simulink model "Force_Att_Controller_Separated"  (R2020a)
settings: Solver=FixedStepAuto  StartTime=0.0  StopTime=20  FixedStep=P.Ts  RelTol=1e-3
PreLoadFcn:
  | parameters
values from neighbouring files (symbols this model uses):
  beta1 = 1    [Run_force_Att_Controller.m]
  kTheta = 0.5/N    (= 0.00333333333333)    [Run_force_Att_Controller.m]
  L = 3    [Run_force_Att_Controller.m]
  m = 3    [Run_force_Att_Controller.m]
  n = length(q)    [Run_force_Att_Controller.m]    (also in circlePoints.m = numberOfPoints)
  N = 150    [Run_force_Att_Controller.m]
  T1 = 1    [Run_force_Att_Controller.m]
  T2 = 0.6    [Run_force_Att_Controller.m]
  ThetaHat0 = [ones(9,1)*1;1]    [Run_force_Att_Controller.m]
  ThetaStar = [0.2061;0.2061;0.2061;0.2061;0.2061;0.2061;6.7315;2.6926;0;1.5]    [Run_force_Att_Controller.m]
  Ts = P.Ts    [Run_force_Att_Controller.m]
  x1_int = [0;-0.15;0.5]    [Run_force_Att_Controller.m]
  x1Dot = [0;0;0]    [Run_force_Att_Controller.m]
  x2_int = [0;0.15;0.5]    [Run_force_Att_Controller.m]
  x2Dot = [0;0;0]    [Run_force_Att_Controller.m]
  xc_int = [0;0;0.5]    [Run_force_Att_Controller.m]
  xcDot = [0;0;0]    [Run_force_Att_Controller.m]
undefined symbols (not defined in the file or in its folder): P
(part 1 of 2)
settings Model: Creator=Daslab  LastModifiedBy=thapa
settings DataIOCC: ReturnWorkspaceOutputs=off
settings DebuggingCC: ArithmeticOperatorsInVariantConditions=warning
settings SFSimCC: SimUseLocalCustomCode=off  CustomCodeUndefinedFunction=UseInterfaceOnly
settings RTWCC: RTWUseLocalCustomCode=off

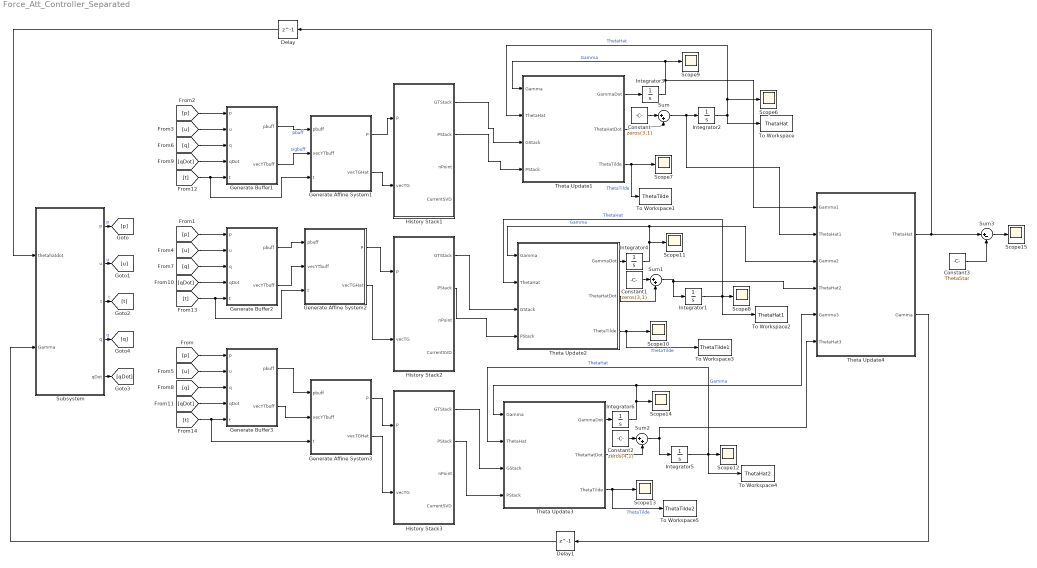
== system Force_Att_Controller_Separated ==
  Constant : Constant  Value=zeros(3,1)
  Constant1 : Constant  Value=zeros(3,1)
  Constant2 : Constant  Value=zeros(4,1)
  Constant3 : Constant  Value=ThetaStar
  Delay : Delay  DelayLength=1  InitialCondition=0
  Delay1 : Delay  DelayLength=1  InitialCondition=0
  Generate Affine System1 : MATLAB Function  TreatAsAtomicUnit=on
  Generate Affine System2 : MATLAB Function  TreatAsAtomicUnit=on
  Generate Affine System3 : MATLAB Function  TreatAsAtomicUnit=on
  Generate Buffer1 : MATLAB Function  TreatAsAtomicUnit=on
  Generate Buffer2 : MATLAB Function  TreatAsAtomicUnit=on
  Generate Buffer3 : MATLAB Function  TreatAsAtomicUnit=on
  History Stack1 : MATLAB Function  TreatAsAtomicUnit=on
  History Stack2 : MATLAB Function  TreatAsAtomicUnit=on
  History Stack3 : MATLAB Function  TreatAsAtomicUnit=on
  Integrator1 : Integrator  InitialCondition=ThetaHat0(4:6,1)
  Integrator2 : Integrator  InitialCondition=ThetaHat0(1:3,1)
  Integrator3 : Integrator  InitialCondition=eye(3)
  Integrator4 : Integrator  InitialCondition=eye(3)
  Integrator5 : Integrator  InitialCondition=ThetaHat0(7:10,1)
  Integrator6 : Integrator  InitialCondition=eye(4)
  Scope{6..15} (10 alike) : Scope
  Subsystem : Subsystem
  Sum : Sum  Inputs=|++
  Sum1 : Sum  Inputs=|++
  Sum2 : Sum  Inputs=|++
  Sum3 : Sum  Inputs=|+-
  Theta Update1 : MATLAB Function  TreatAsAtomicUnit=on
  Theta Update2 : MATLAB Function  TreatAsAtomicUnit=on
  Theta Update3 : MATLAB Function  TreatAsAtomicUnit=on
  Theta Update4 : MATLAB Function  TreatAsAtomicUnit=on
  To Workspace : ToWorkspace  VariableName=ThetaHat  SaveFormat=Timeseries  SampleTime=-1
  To Workspace1 : ToWorkspace  VariableName=ThetaTilde  SaveFormat=Timeseries  SampleTime=-1
  To Workspace2 : ToWorkspace  VariableName=ThetaHat1  SaveFormat=Timeseries  SampleTime=-1
  To Workspace3 : ToWorkspace  VariableName=ThetaTilde1  SaveFormat=Timeseries  SampleTime=-1
  To Workspace4 : ToWorkspace  VariableName=ThetaHat2  SaveFormat=Timeseries  SampleTime=-1
  To Workspace5 : ToWorkspace  VariableName=ThetaTilde2  SaveFormat=Timeseries  SampleTime=-1
  wires:
  Theta Update1/3(ThetaTilde) -> Scope7/1, To Workspace1/1  "ThetaTilde"
  History Stack1/1(GTStack) -> Theta Update1/3(GStack)
  Generate Affine System1/1(P) -> History Stack1/1(P)
  Integrator2/1 -> Scope6/1, Theta Update1/2(ThetaHat), To Workspace/1  "ThetaHat"
  History Stack1/2(PStack) -> Theta Update1/4(PStack)
  Integrator3/1 -> Scope9/1, Theta Update1/1(Gamma), Theta Update4/1(Gamma1)  "Gamma"
  Theta Update1/1(GammaDot) -> Integrator3/1
  Constant/1 -> Sum/1
  Sum/1 -> Theta Update4/2(ThetaHat1), Integrator2/1
  Theta Update1/2(ThetaHatDot) -> Sum/2
  Delay/1 -> Subsystem/1(thetahatdot)
  Generate Buffer1/1(pbuff) -> Generate Affine System1/1(pbuff)  "pbuff"
  Generate Buffer1/2(vecYTbuff) -> Generate Affine System1/2(vecYTbuff)  "sigbuff"
  Generate Affine System1/2(vecTGHat) -> History Stack1/2(vecTG)
  History Stack2/1(GTStack) -> Theta Update2/3(GStack)
  History Stack2/2(PStack) -> Theta Update2/4(PStack)
  History Stack3/1(GTStack) -> Theta Update3/3(GStack)
  History Stack3/2(PStack) -> Theta Update3/4(PStack)
  Sum1/1 -> Theta Update4/4(ThetaHat2), Integrator1/1
  Theta Update2/2(ThetaHatDot) -> Sum1/2
  Integrator4/1 -> Scope11/1, Theta Update4/3(Gamma2), Theta Update2/1(Gamma)  "Gamma"
  Constant1/1 -> Sum1/1
  Integrator1/1 -> Theta Update2/2(ThetaHat), Scope8/1, To Workspace2/1  "ThetaHat"
  Theta Update2/3(ThetaTilde) -> Scope10/1, To Workspace3/1  "ThetaTilde"
  Theta Update2/1(GammaDot) -> Integrator4/1
  Sum2/1 -> Theta Update4/6(ThetaHat3), Integrator5/1
  Theta Update3/2(ThetaHatDot) -> Sum2/2
  Integrator6/1 -> Scope14/1, Theta Update3/1(Gamma), Theta Update4/5(Gamma3)  "Gamma"
  Constant2/1 -> Sum2/1
  Integrator5/1 -> Theta Update3/2(ThetaHat), Scope12/1, To Workspace4/1  "ThetaHat"
  Theta Update3/3(ThetaTilde) -> Scope13/1, To Workspace5/1  "ThetaTilde"
  Theta Update3/1(GammaDot) -> Integrator6/1
  Generate Affine System3/1(P) -> History Stack3/1(P)
  Generate Affine System3/2(vecTGHat) -> History Stack3/2(vecTG)
  Generate Affine System2/1(P) -> History Stack2/1(P)
  Generate Affine System2/2(vecTGHat) -> History Stack2/2(vecTG)
  Generate Buffer2/1(pbuff) -> Generate Affine System2/1(pbuff)
  Generate Buffer2/2(vecYTbuff) -> Generate Affine System2/2(vecYTbuff)
  Generate Buffer3/1(pbuff) -> Generate Affine System3/1(pbuff)
  Generate Buffer3/2(vecYTbuff) -> Generate Affine System3/2(vecYTbuff)
  Theta Update4/2(Gamma) -> Delay1/1
  Delay1/1 -> Subsystem/2(Gamma)
  Theta Update4/1(ThetaHat) -> Sum3/1, Delay/1
  Constant3/1 -> Sum3/2
  Sum3/1 -> Scope15/1
  Subsystem/1(p) -> [p]  "p"
  [p] -> Generate Buffer1/1(p)
  Subsystem/2(u) -> [u]  "u"
  Subsystem/5(qDot) -> [qDot]
  Subsystem/4(q) -> [q]  "q"
  Subsystem/3(t) -> [t]  "t"
  [p] -> Generate Buffer2/1(p)
  [p] -> Generate Buffer3/1(p)
  [u] -> Generate Buffer1/2(u)
  [u] -> Generate Buffer2/2(u)
  [u] -> Generate Buffer3/2(u)
  [q] -> Generate Buffer1/3(q)
  [q] -> Generate Buffer2/3(q)
  [q] -> Generate Buffer3/3(q)
  [qDot] -> Generate Buffer1/4(qDot)
  [qDot] -> Generate Buffer2/4(qDot)
  [qDot] -> Generate Buffer3/4(qDot)
  [t] -> Generate Affine System1/3(t), Generate Buffer1/5(t)
  [t] -> Generate Affine System2/3(t), Generate Buffer2/5(t)
  [t] -> Generate Affine System3/3(t), Generate Buffer3/5(t)

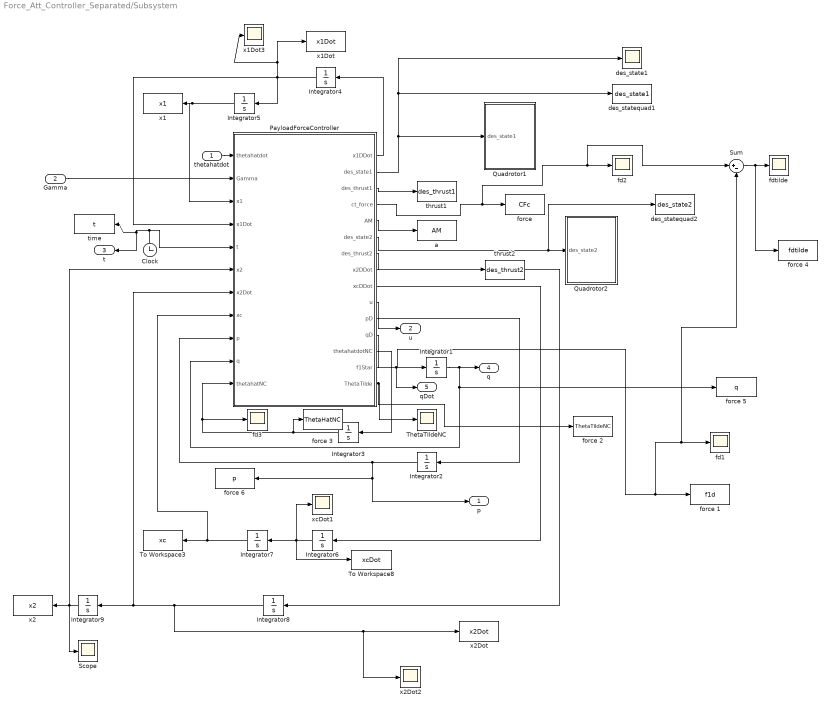
== system Force_Att_Controller_Separated/Subsystem ==
  thetahatdot : Inport
  Gamma : Inport  Port=2
  Clock : Clock
  Integrator1 : Integrator  InitialCondition=[x1Dot;x2Dot;xcDot]
  Integrator2 : Integrator  InitialCondition=[x1_int;x2_int;xc_int]
  Integrator3 : Integrator  InitialCondition=ones(10,1)
  Integrator4 : Integrator  InitialCondition=x1Dot
  Integrator5 : Integrator  InitialCondition=x1_int
  Integrator6 : Integrator  InitialCondition=xcDot
  Integrator7 : Integrator  InitialCondition=xc_int
  Integrator8 : Integrator  InitialCondition=x2Dot
  Integrator9 : Integrator  InitialCondition=x2_int
  PayloadForceController : MATLAB Function  TreatAsAtomicUnit=on
  Quadrotor1 : Subsystem
  Quadrotor2 : Subsystem
  Scope : Scope
  Sum : Sum  Inputs=|+-
  ThetaTIldeNC : Scope
  To Workspace3 : ToWorkspace  VariableName=xc  SampleTime=-1
  To Workspace8 : ToWorkspace  VariableName=xcDot  SampleTime=-1
  "a " : ToWorkspace  VariableName=AM  SampleTime=-1
  des_state1 : Scope
  "des_statequad1 " : ToWorkspace  VariableName=des_state1  SampleTime=-1
      settings: Save2DSignal=2-D array (concatenate along first dimension)
  des_statequad2 : ToWorkspace  VariableName=des_state2  SampleTime=-1
      settings: Save2DSignal=2-D array (concatenate along first dimension)
  fd1 : Scope
  fd2 : Scope
  fd3 : Scope
  fdtilde : Scope
  "force " : ToWorkspace  VariableName=CFc  SampleTime=-1
  force 1 : ToWorkspace  VariableName=f1d  SampleTime=-1
  force 2 : ToWorkspace  VariableName=ThetaTildeNC  SampleTime=-1
  force 3 : ToWorkspace  VariableName=ThetaHatNC  SampleTime=-1
  force 4 : ToWorkspace  VariableName=fdtilde  SampleTime=-1
  force 5 : ToWorkspace  VariableName=q  SampleTime=-1
      settings: Save2DSignal=2-D array (concatenate along first dimension)
  force 6 : ToWorkspace  VariableName=p  SampleTime=-1
      settings: Save2DSignal=2-D array (concatenate along first dimension)
  thrust1 : ToWorkspace  VariableName=des_thrust1  SampleTime=-1
      settings: Save2DSignal=2-D array (concatenate along first dimension)
  thrust2 : ToWorkspace  VariableName=des_thrust2  SampleTime=-1
  time : ToWorkspace  VariableName=t  SampleTime=-1
  x1 : ToWorkspace  VariableName=x1  SampleTime=-1
  x1Dot : ToWorkspace  VariableName=x1Dot  SampleTime=-1
  x1Dot3 : Scope
  x2 : ToWorkspace  VariableName=x2  SampleTime=-1
  x2Dot : ToWorkspace  VariableName=x2Dot  SampleTime=-1
  x2Dot2 : Scope
  xcDot1 : Scope
  p : Outport  VectorParamsAs1DForOutWhenUnconnected=off
  u : Outport  Port=2  VectorParamsAs1DForOutWhenUnconnected=off
  t : Outport  Port=3  VectorParamsAs1DForOutWhenUnconnected=off
  q : Outport  Port=4  VectorParamsAs1DForOutWhenUnconnected=off
  qDot : Outport  Port=5  VectorParamsAs1DForOutWhenUnconnected=off
  wires:
  PayloadForceController/7(des_thrust2) -> thrust2/1
  Integrator6/1 -> Integrator7/1, xcDot1/1, To Workspace8/1
  PayloadForceController/4(ct_force) -> Sum/1, fd2/1, "force "/1
  PayloadForceController/9(xcDDot) -> Integrator6/1
  PayloadForceController/5(AM) -> "a "/1
  PayloadForceController/2(des_state1) -> "des_statequad1 "/1, des_state1/1, Quadrotor1/1(des_state1)
  PayloadForceController/3(des_thrust1) -> thrust1/1
  Clock/1 -> time/1, t/1, PayloadForceController/5(t)
  Integrator7/1 -> PayloadForceController/8(xc), To Workspace3/1
  Integrator8/1 -> PayloadForceController/7(x2Dot), Integrator9/1, x2Dot2/1, x2Dot/1
  PayloadForceController/1(x1DDot) -> Integrator4/1
  Integrator4/1 -> Integrator5/1, x1Dot3/1, x1Dot/1, PayloadForceController/4(x1Dot)
  Integrator9/1 -> Scope/1, PayloadForceController/6(x2), x2/1
  Integrator5/1 -> PayloadForceController/3(x1), x1/1
  PayloadForceController/6(des_state2) -> des_statequad2/1, Quadrotor2/1(des_state2)
  PayloadForceController/8(x2DDot) -> Integrator8/1
  PayloadForceController/10(u) -> u/1
  Integrator1/1 -> PayloadForceController/10(q), force 5/1, q/1
  Integrator2/1 -> p/1, force 6/1, PayloadForceController/9(p)
  PayloadForceController/11(pD) -> Integrator2/1
  PayloadForceController/12(qD) -> qDot/1, Integrator1/1
  thetahatdot/1 -> PayloadForceController/1(thetahatdot)
  PayloadForceController/13(thetahatdotNC) -> Integrator3/1
  Integrator3/1 -> force 3/1, PayloadForceController/11(thetahatNC), fd3/1
  Gamma/1 -> PayloadForceController/2(Gamma)
  PayloadForceController/14(f1Star) -> Sum/2, fd1/1, force 1/1
  PayloadForceController/15(ThetaTilde) -> force 2/1, ThetaTIldeNC/1
  Sum/1 -> force 4/1, fdtilde/1

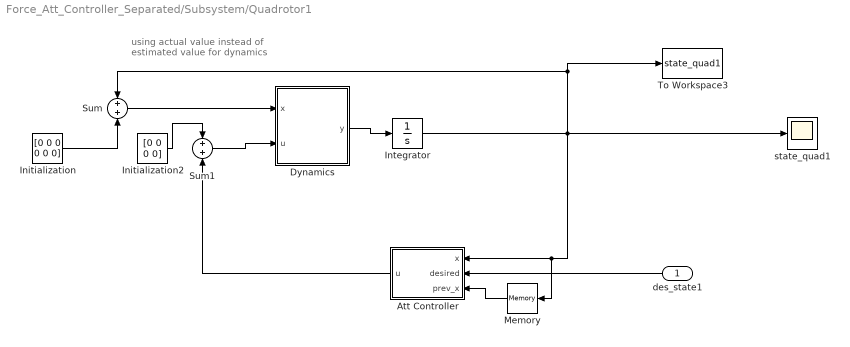
== system Force_Att_Controller_Separated/Subsystem/Quadrotor1 ==
  note: using actual value instead of estimated value for dynamics
  des_state1 : Inport
  Att Controller : MATLAB Function  TreatAsAtomicUnit=on
  Dynamics : MATLAB Function  TreatAsAtomicUnit=on  SystemSampleTime=P.Ts
  Initialization : Constant  Value=[0 0 0 0 0 0]
  Initialization2 : Constant  Value=[0 0 0 0]
  Integrator : Integrator
  Memory : Memory  InitialCondition=[0 0 0 0 0 0]
  Sum : Sum
  Sum1 : Sum
  To Workspace3 : ToWorkspace  VariableName=state_quad1  SampleTime=-1
      settings: Save2DSignal=2-D array (concatenate along first dimension)
  state_quad1 : Scope
  wires:
  Memory/1 -> Att Controller/3(prev_x)
  Initialization2/1 -> Sum1/1
  Att Controller/1(u) -> Sum1/2
  Dynamics/1(y) -> Integrator/1
  Initialization/1 -> Sum/2
  Integrator/1 -> Memory/1, Att Controller/1(x), state_quad1/1, Sum/1, To Workspace3/1
  Sum1/1 -> Dynamics/2(u)
  Sum/1 -> Dynamics/1(x)
  des_state1/1 -> Att Controller/2(desired)

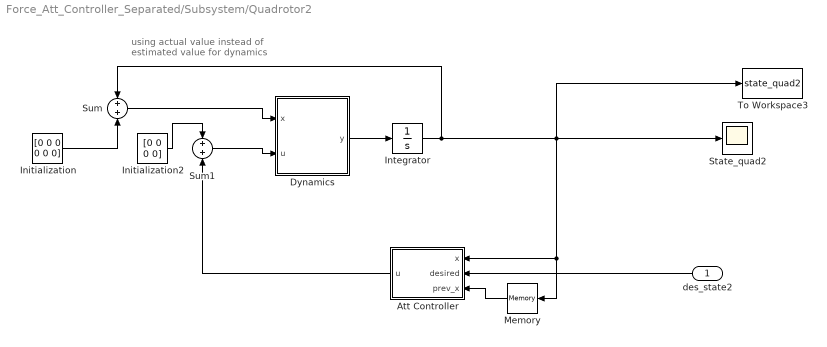
== system Force_Att_Controller_Separated/Subsystem/Quadrotor2 ==
  note: using actual value instead of estimated value for dynamics
  des_state2 : Inport
  Att Controller : MATLAB Function  TreatAsAtomicUnit=on
  Dynamics : MATLAB Function  TreatAsAtomicUnit=on  SystemSampleTime=P.Ts
  Initialization : Constant  Value=[0 0 0 0 0 0]
  Initialization2 : Constant  Value=[0 0 0 0]
  Integrator : Integrator
  Memory : Memory  InitialCondition=[0 0 0 0 0 0]
  State_quad2 : Scope
  Sum : Sum
  Sum1 : Sum
  To Workspace3 : ToWorkspace  VariableName=state_quad2  SampleTime=-1
      settings: Save2DSignal=2-D array (concatenate along first dimension)
  wires:
  Memory/1 -> Att Controller/3(prev_x)
  Initialization2/1 -> Sum1/1
  Att Controller/1(u) -> Sum1/2
  Dynamics/1(y) -> Integrator/1
  Initialization/1 -> Sum/2
  Integrator/1 -> State_quad2/1, Memory/1, Att Controller/1(x), To Workspace3/1, Sum/1
  Sum1/1 -> Dynamics/2(u)
  Sum/1 -> Dynamics/1(x)
  des_state2/1 -> Att Controller/2(desired)

== matlab function Force_Att_Controller_Separated/Subsystem/Quadrotor2/Dynamics ==
  data: x input; u input; y output; P parameter
function y = fcn(x, u, P)
%#codegen
%References: Quadrotor Dynamics and Control Rev 0.1
%Randal Beard

%A Simple Attitude Control of Quadrotor Helicopter Based on
%Ziegler-Nichols Rules for Tuning PD Parameters
%ZeFang He and Long Zhao

wind = [0 0 0]';

m = P.m;
g = P.g;
Ix = P.Ix;
Iy = P.Iy;
Iz = P.Iz;
L = P.L;

Cd = zeros(3,1);
Cd(1:3) = P.Cd1 + 0.9*exp(-0.6*(norm(wind(1:3)+x(4:6))-2));


% Cd = zeros(3,1);
% Cd(1) = P.Cd1 + 0.9*exp(-0.6*(abs(wind(1)+x(4)) - 2));
% Cd(2) = P.Cd2 + 0.9*exp(-0.6*(abs(wind(2)+x(5)) - 2));
% Cd(3) = P.Cd3 + 0.9*exp(-0.6*(abs(wind(3)+x(6)) - 2));
for i=1:3
    if Cd(i) > 1.1
        Cd(i) = 1.1;
    end
end

y = x;

%Calculate drag force on quadrotor
mag_V = wind + x(4:6);
%mag_V = x(4:6);
mag_Combined = norm(mag_V); %airspeed magnitude
force = Cd * mag_Combined^2;

Fw = zeros(3,1);
if mag_Combined ~= 0
    Fw = diag(mag_V/mag_Combined) * force;
else
    Fw(:) = 0;
end

% y(1) = -x(4) + wind(1);
% y(2) = -x(5) + (wind(2));
% y(3) = -x(6) + (wind(3));
%y(1) = 0;%-x(4);
%y(2) = 0;%-x(5);
%y(3) = 0;%-x(6);
%y(4) = 0;%(u(1))/m*(cos(x(7))*sin(x(8))*cos(x(9)) +...
    %sin(x(7))*sin(x(9))) + Fw(1)/m;%1/m*sign(x(4))*Cd1*x(4)^2;
%y(5) = 0;%-(u(1))/m*(+cos(x(7))*sin(x(8))*sin(x(9)) -...
    %sin(x(7))*cos(x(9))) + Fw(2)/m;%1/m*sign(x(5))*Cd2*x(5)^2;
%y(6) = 0;%g - (u(1))/m*(cos(x(7)) * cos(x(8))) + Fw(3);%1/m*sign(x(6))*Cd3*x(5)^2;

%roll, pitch, yaw: phi, theta, psi
y(1) = x(4);
y(2) = x(5);
y(3) = x(6);
y(4) = x(5)*x(6)*(Iy-Iz)/Ix + 1/Ix*u(2);
y(5) = x(4)*x(6)*(Iz-Ix)/Iy + 1/Iy*u(3);
y(6) = x(4)*x(5)*(Ix - Iy)/Iz + u(4)/Iz;

== matlab function Force_Att_Controller_Separated/Generate Buffer2 ==
  settings: updateMethod=DISCRETE  sampleTime=Ts
  data: pbuff output; p input; u input; q input; qDot input; t input; T1 parameter; T2 parameter; Ts parameter; n parameter; L parameter; vecYTbuff output; P parameter
function [pbuff,vecYTbuff] = fcn(p,u,q,qDot,t,T1,T2,Ts,n,L,P)
%#codegen
persistent PTemp sigTemp;
if isempty(PTemp)
    PTemp = 0*ones(n/3,round((T1)/Ts)+1); % initalize the persistent variable
end

if isempty(sigTemp)
    sigTemp = zeros(n/3*L,round((T1)/Ts)+1);
end
% Known part of the system dynamics
qDotbuff = zeros(9,1);
x1 = p(1:3,1);
x2 = p(4:6,1);
xc = p(7:9,1);
x1Dot = q(1:3,1);
x2Dot = q(4:6,1);
xcDot = q(7:9,1);
m1 = P.m;
m2 = m1;
Mc = P.Mc;
g = P.g;
k = P.k;

e3 = [0 0 1]';

R_theta = eye(3,3);     

r1 = [0 -0.15 0]';
r2 = [0 0.15 0]';

a1 = xc + R_theta*r1; 

a2 = xc + R_theta*r2;

z1 = x1 - a1;

z2 = x2 - a2;

f1 = k*z1;  % linear model 

f2 = k*z2;   % linear model 


fo = [(u(4:6,1) - f2 - m2*g*e3)/m2];

Y_N = diag([1/m2*norm(x2Dot)*x2Dot]);
Y_c = [eye(3),qDot(7:9,1) + g*e3];


Y = [Y_N];
 
qDotbuff(1:6,1) = qDot(1:6,1);
qDotbuff(7:9,1) = zeros(3,1);

sig = reshape(Y.',n/3*L,1);

PPP=PTemp(:,2:end);
SSS=sigTemp(:,2:end);
PTemp=[PPP fo-qDotbuff(4:6,1)];
sigTemp=[SSS sig];
pbuff=PTemp;
vecYTbuff=sigTemp;

== matlab function Force_Att_Controller_Separated/Generate Affine System2 ==
  data: P output; pbuff input; vecYTbuff input; t input; Ts parameter; T2 parameter; T1 parameter; vecTGHat output
function [P,vecTGHat]  = fcn(pbuff,vecYTbuff,t ,Ts, T2, T1)
%#codegen
T1Round=round(T1/Ts);

P1=pbuff(:,end-T1Round:end);
G1=vecYTbuff(:,end-T1Round:end);

P = (t>T1)*Ts*trapz(P1,2);
vecTGHat = (t>T1)*Ts*trapz(G1,2);

== matlab function Force_Att_Controller_Separated/Subsystem/Quadrotor1/Dynamics ==
  data: x input; u input; y output; P parameter
function y = fcn(x, u, P)
%#codegen
%References: Quadrotor Dynamics and Control Rev 0.1
%Randal Beard

%A Simple Attitude Control of Quadrotor Helicopter Based on
%Ziegler-Nichols Rules for Tuning PD Parameters
%ZeFang He and Long Zhao

wind = [0 0 0]';

m = P.m;
g = P.g;
Ix = P.Ix;
Iy = P.Iy;
Iz = P.Iz;
L = P.L;

Cd = zeros(3,1);
Cd(1:3) = P.Cd1 + 0.9*exp(-0.6*(norm(wind(1:3)+x(4:6))-2));


% Cd = zeros(3,1);
% Cd(1) = P.Cd1 + 0.9*exp(-0.6*(abs(wind(1)+x(4)) - 2));
% Cd(2) = P.Cd2 + 0.9*exp(-0.6*(abs(wind(2)+x(5)) - 2));
% Cd(3) = P.Cd3 + 0.9*exp(-0.6*(abs(wind(3)+x(6)) - 2));
for i=1:3
    if Cd(i) > 1.1
        Cd(i) = 1.1;
    end
end

y = x;

%Calculate drag force on quadrotor
mag_V = wind + x(4:6);
%mag_V = x(4:6);
mag_Combined = norm(mag_V); %airspeed magnitude
force = Cd * mag_Combined^2;

Fw = zeros(3,1);
if mag_Combined ~= 0
    Fw = diag(mag_V/mag_Combined) * force;
else
    Fw(:) = 0;
end

% y(1) = -x(4) + wind(1);
% y(2) = -x(5) + (wind(2));
% y(3) = -x(6) + (wind(3));
%y(1) = 0;%-x(4);
%y(2) = 0;%-x(5);
%y(3) = 0;%-x(6);
%y(4) = 0;%(u(1))/m*(cos(x(7))*sin(x(8))*cos(x(9)) +...
    %sin(x(7))*sin(x(9))) + Fw(1)/m;%1/m*sign(x(4))*Cd1*x(4)^2;
%y(5) = 0;%-(u(1))/m*(+cos(x(7))*sin(x(8))*sin(x(9)) -...
    %sin(x(7))*cos(x(9))) + Fw(2)/m;%1/m*sign(x(5))*Cd2*x(5)^2;
%y(6) = 0;%g - (u(1))/m*(cos(x(7)) * cos(x(8))) + Fw(3);%1/m*sign(x(6))*Cd3*x(5)^2;

%roll, pitch, yaw: phi, theta, psi
y(1) = x(4);
y(2) = x(5);
y(3) = x(6);
y(4) = x(5)*x(6)*(Iy-Iz)/Ix + 1/Ix*u(2);
y(5) = x(4)*x(6)*(Iz-Ix)/Iy + 1/Iy*u(3);
y(6) = x(4)*x(5)*(Ix - Iy)/Iz + u(4)/Iz;

== matlab function Force_Att_Controller_Separated/History Stack2 ==
  settings: updateMethod=DISCRETE  sampleTime=Ts
  data: P input; GTStack output; vecTG input; N parameter; n parameter; L parameter; PStack output; nPoint output; CurrentSVD output
function [GTStack,PStack,nPoint,CurrentSVD] =...
    fcn(P,vecTG, N, n, L )
%#codegen,FStackStored, GStackStored, PStackStored
persistent GStackHPersist PStackHPersist nPoints eta;
% if isempty(FStackHPersist)
% %    FStackHPersist = FStackStored; % initalize the persistent variable
%      FStackHPersist = zeros(n,N);
% end
if isempty(GStackHPersist)
 %   GStackHPersist = GStackStored;
    GStackHPersist = zeros(L,n/3*N);
end
if isempty(PStackHPersist)
%    PStackHPersist = PStackStored;
     PStackHPersist = zeros(n/3,N);
end
if isempty(nPoints)
    nPoints = 0;
end
if isempty(eta)
    eta = 0;
end
%GHatTStack is [intY1' intY2' ... intYN']
%FHatStack is [FHat1 FHat2 ... FHatN]
%and so is PStack
G = (reshape(vecTG,L,n/3)).';

%Operations 
CurrentScriptH = GStackHPersist*GStackHPersist';
CurrentSingularValue = min(svd(CurrentScriptH));
SingularValueList = zeros(N,1);
for i=1:N
    ithGTranspose = GStackHPersist(:,(i-1)*n/3+1:i*n/3);
    NewScriptH = CurrentScriptH + G'*G...
        -ithGTranspose*ithGTranspose';
    SingularValueList(i,1)=min(svd(NewScriptH));
end

[NewSingularValue,ind]=max(SingularValueList);
%Update persistent variables
if NewSingularValue>CurrentSingularValue + 0*CurrentSingularValue
    GStackHPersist(:,(ind-1)*n/3+1:ind*n/3) = G';
    %FStackHPersist(:,ind) = FHat;
    PStackHPersist(:,ind) = P;
    nPoints = nPoints+1;
end
if NewSingularValue>eta
    eta=NewSingularValue;
end
%Output
CurrentSVD = min(svd(GStackHPersist*GStackHPersist'));
%FStack=FStackHPersist;
GTStack=GStackHPersist;
PStack=PStackHPersist;
nPoint = nPoints;



% 

% 
% 
% persistent FStackHPersist GStackHPersist PStackHPersist FStackGPersist GStackGPersist PStackGPersist nPoints nPurges eta;
% if isempty(FStackHPersist)
%     FStackHPersist = zeros(n,N); % initalize the persistent variable
% end
% if isempty(GStackHPersist)
%     GStackHPersist = zeros(L,n*N);
% end
% if isempty(PStackHPersist)
%     PStackHPersist = zeros(n,N);
% end
% if isempty(FStackGPersist)
%     FStackGPersist = zeros(n,N); % initalize the persistent variable
% end
% if isempty(GStackGPersist)
%     GStackGPersist = zeros(L,n*N);
% end
% if isempty(PStackGPersist)
%     PStackGPersist = zeros(n,N);
% end
% if isempty(nPoints)
%     nPoints = 0;
% end
% if isempty(nPurges)
%     nPurges = 0;
% end
% if isempty(eta)
%     eta = 0;
% end
% %GHatTStack is [intY1' intY2' ... intYN']
% %FHatStack is [FHat1 FHat2 ... FHatN]
% %and so is PStack
% GHat = (reshape(vecTG,L,n)).';
% 
% %Operations 
% CurrentScriptG = GStackGPersist*GStackGPersist';
% CurrentSingularValue = min(svd(CurrentScriptG));
% SingularValueList = zeros(N,1);
% for i=1:N
%     ithGTranspose = GStackGPersist(:,(i-1)*n+1:i*n);
%     NewScriptG = CurrentScriptG + GHat'*GHat...
%         -ithGTranspose*ithGTranspose';
%     SingularValueList(i,1)=min(svd(NewScriptG));
% end
% [NewSingularValue,ind]=max(SingularValueList);
% %Update persistent variables
% if NewSingularValue>CurrentSingularValue + 0*CurrentSingularValue
%     GStackGPersist(:,(ind-1)*n+1:ind*n) = GHat';
%     FStackGPersist(:,ind) = FHat;
%     PStackGPersist(:,ind) = P;
%     nPoints = nPoints+1;
% end
% if nPurges==0
%     FStackHPersist=FStackGPersist;
% end
% if nPoints >= N && NewSingularValue>0.95*eta
%     nPoints = 0;
%     FStackHPersist = FStackGPersist;
%     FStackGPersist = zeros(n,N);
%     GStackHPersist = GStackGPersist;
%     GStackGPersist = zeros(L,n*N);
%     PStackHPersist = PStackGPersist;
%     PStackGPersist = zeros(n,N);
%     nPurges = nPurges+1;
% end
% if NewSingularValue>eta
%     eta=NewSingularValue;
% end
% %Output
% CurrentSVD = min(svd(GStackHPersist*GStackHPersist'));
% FStack=FStackHPersist;
% GTStack=GStackHPersist;
% PStack=PStackHPersist;
% nPoint = nPoints;
% nPurge = nPurges;

== matlab function Force_Att_Controller_Separated/Generate Affine System1 ==
  data: P output; pbuff input; vecYTbuff input; t input; Ts parameter; T2 parameter; T1 parameter; vecTGHat output
function [P,vecTGHat]  = fcn(pbuff,vecYTbuff,t ,Ts, T2, T1)
%#codegen
T1Round=round(T1/Ts);

P1=pbuff(:,end-T1Round:end);
G1=vecYTbuff(:,end-T1Round:end);

P = (t>T1)*Ts*trapz(P1,2);
vecTGHat = (t>T1)*Ts*trapz(G1,2);

== matlab function Force_Att_Controller_Separated/Generate Buffer1 ==
  settings: updateMethod=DISCRETE  sampleTime=Ts
  data: pbuff output; p input; u input; q input; qDot input; t input; T1 parameter; T2 parameter; Ts parameter; n parameter; L parameter; vecYTbuff output; P parameter
function [pbuff,vecYTbuff] = fcn(p,u,q,qDot,t,T1,T2,Ts,n,L,P)
%#codegen
persistent PTemp sigTemp;
if isempty(PTemp)
    PTemp = 0*ones(n/3,round((T1)/Ts)+1); % initalize the persistent variable
end

if isempty(sigTemp)
    sigTemp = zeros(n/3*L,round((T1)/Ts)+1);
end
% Known part of the system dynamics
qDotbuff = zeros(9,1);
x1 = p(1:3,1);
x2 = p(4:6,1);
xc = p(7:9,1);
x1Dot = q(1:3,1);
x2Dot = q(4:6,1);
xcDot = q(7:9,1);
m1 = P.m;
m2 = m1;
Mc = P.Mc;
g = P.g;
k = P.k;

e3 = [0 0 1]';

R_theta = eye(3,3);     

r1 = [0 -0.15 0]';
r2 = [0 0.15 0]';

a1 = xc + R_theta*r1; 

a2 = xc + R_theta*r2;

z1 = x1 - a1;

z2 = x2 - a2;

f1 = k*z1;  % linear model 

f2 = k*z2;   % linear model 


fo = [(u(1:3,1) - f1 - m1*g*e3)/m1];

Y_N = diag([1/m1*norm(x1Dot)*x1Dot]);
Y_c = [eye(3),qDot(7:9,1) + g*e3];


Y = [Y_N];
 
qDotbuff(1:6,1) = qDot(1:6,1);
qDotbuff(7:9,1) = zeros(3,1);

sig = reshape(Y.',n/3*L,1);

PPP=PTemp(:,2:end);
SSS=sigTemp(:,2:end);
PTemp=[PPP fo-qDotbuff(1:3,1)];
sigTemp=[SSS sig];
pbuff=PTemp;
vecYTbuff=sigTemp;

== matlab function Force_Att_Controller_Separated/History Stack1 ==
  settings: updateMethod=DISCRETE  sampleTime=Ts
  data: P input; GTStack output; vecTG input; N parameter; n parameter; L parameter; PStack output; nPoint output; CurrentSVD output
function [GTStack,PStack,nPoint,CurrentSVD] =...
    fcn(P,vecTG, N, n, L )
%#codegen,FStackStored, GStackStored, PStackStored
persistent GStackHPersist PStackHPersist nPoints eta;
% if isempty(FStackHPersist)
% %    FStackHPersist = FStackStored; % initalize the persistent variable
%      FStackHPersist = zeros(n,N);
% end
if isempty(GStackHPersist)
 %   GStackHPersist = GStackStored;
    GStackHPersist = zeros(L,n/3*N);
end
if isempty(PStackHPersist)
%    PStackHPersist = PStackStored;
     PStackHPersist = zeros(n/3,N);
end
if isempty(nPoints)
    nPoints = 0;
end
if isempty(eta)
    eta = 0;
end
%GHatTStack is [intY1' intY2' ... intYN']
%FHatStack is [FHat1 FHat2 ... FHatN]
%and so is PStack
G = (reshape(vecTG,L,n/3)).';

%Operations 
CurrentScriptH = GStackHPersist*GStackHPersist';
CurrentSingularValue = min(svd(CurrentScriptH));
SingularValueList = zeros(N,1);
for i=1:N
    ithGTranspose = GStackHPersist(:,(i-1)*n/3+1:i*n/3);
    NewScriptH = CurrentScriptH + G'*G...
        -ithGTranspose*ithGTranspose';
    SingularValueList(i,1)=min(svd(NewScriptH));
end

[NewSingularValue,ind]=max(SingularValueList);
%Update persistent variables
if NewSingularValue>CurrentSingularValue + 0*CurrentSingularValue
    GStackHPersist(:,(ind-1)*n/3+1:ind*n/3) = G';
    %FStackHPersist(:,ind) = FHat;
    PStackHPersist(:,ind) = P;
    nPoints = nPoints+1;
end
if NewSingularValue>eta
    eta=NewSingularValue;
end
%Output
CurrentSVD = min(svd(GStackHPersist*GStackHPersist'));
%FStack=FStackHPersist;
GTStack=GStackHPersist;
PStack=PStackHPersist;
nPoint = nPoints;



% 

% 
% 
% persistent FStackHPersist GStackHPersist PStackHPersist FStackGPersist GStackGPersist PStackGPersist nPoints nPurges eta;
% if isempty(FStackHPersist)
%     FStackHPersist = zeros(n,N); % initalize the persistent variable
% end
% if isempty(GStackHPersist)
%     GStackHPersist = zeros(L,n*N);
% end
% if isempty(PStackHPersist)
%     PStackHPersist = zeros(n,N);
% end
% if isempty(FStackGPersist)
%     FStackGPersist = zeros(n,N); % initalize the persistent variable
% end
% if isempty(GStackGPersist)
%     GStackGPersist = zeros(L,n*N);
% end
% if isempty(PStackGPersist)
%     PStackGPersist = zeros(n,N);
% end
% if isempty(nPoints)
%     nPoints = 0;
% end
% if isempty(nPurges)
%     nPurges = 0;
% end
% if isempty(eta)
%     eta = 0;
% end
% %GHatTStack is [intY1' intY2' ... intYN']
% %FHatStack is [FHat1 FHat2 ... FHatN]
% %and so is PStack
% GHat = (reshape(vecTG,L,n)).';
% 
% %Operations 
% CurrentScriptG = GStackGPersist*GStackGPersist';
% CurrentSingularValue = min(svd(CurrentScriptG));
% SingularValueList = zeros(N,1);
% for i=1:N
%     ithGTranspose = GStackGPersist(:,(i-1)*n+1:i*n);
%     NewScriptG = CurrentScriptG + GHat'*GHat...
%         -ithGTranspose*ithGTranspose';
%     SingularValueList(i,1)=min(svd(NewScriptG));
% end
% [NewSingularValue,ind]=max(SingularValueList);
% %Update persistent variables
% if NewSingularValue>CurrentSingularValue + 0*CurrentSingularValue
%     GStackGPersist(:,(ind-1)*n+1:ind*n) = GHat';
%     FStackGPersist(:,ind) = FHat;
%     PStackGPersist(:,ind) = P;
%     nPoints = nPoints+1;
% end
% if nPurges==0
%     FStackHPersist=FStackGPersist;
% end
% if nPoints >= N && NewSingularValue>0.95*eta
%     nPoints = 0;
%     FStackHPersist = FStackGPersist;
%     FStackGPersist = zeros(n,N);
%     GStackHPersist = GStackGPersist;
%     GStackGPersist = zeros(L,n*N);
%     PStackHPersist = PStackGPersist;
%     PStackGPersist = zeros(n,N);
%     nPurges = nPurges+1;
% end
% if NewSingularValue>eta
%     eta=NewSingularValue;
% end
% %Output
% CurrentSVD = min(svd(GStackHPersist*GStackHPersist'));
% FStack=FStackHPersist;
% GTStack=GStackHPersist;
% PStack=PStackHPersist;
% nPoint = nPoints;
% nPurge = nPurges;

== matlab function Force_Att_Controller_Separated/Theta Update1 ==
  data: Gamma input; GammaDot output; ThetaHat input; GStack input; PStack input; N parameter; n parameter; m parameter; ThetaHatDot output; kTheta parameter; beta1 parameter; ThetaStar parameter; ThetaTilde output
function [GammaDot,ThetaHatDot,ThetaTilde]  = fcn(Gamma,ThetaHat,...
    GStack,PStack,N,n,m,kTheta, beta1, ThetaStar)
%#codegen
% persistent persistThetaHatDot
% if isempty(persistThetaHatDot)
%     persistThetaHatDot = zeros(10,1);
% end
%CaligraphicGStack is [CaligraphicG1' CaligraphicG2' ... CaligraphicGN']
%CaligraphicFStack is [CaligraphicF1 CaligraphicF2 ... CaligraphicFN]
alpha = 0.01;
% Gamma1 = Gamma(1:3,1:3);
% Gamma2 = Gamma(4:6,4:6);
% Gamma3 = Gamma(7:10,7:10);
% ThetaHat1 = ThetaHat(1:3,1);
% ThetaHat2 = ThetaHat(4:6,1);
% ThetaHat3 = ThetaHat(7:10,1);
ThetaHatDot = kTheta*Gamma*(GStack*...
    (reshape(PStack,n/3*N,1)-GStack'*ThetaHat));
% ThetaHatDot2 = kTheta*Gamma2*(GStack(4:6,3*N+1:6*N)*...
%     (reshape(PStack(4:6,:),3*N,1)-GStack(4:6,3*N+1:6*N)'*ThetaHat2));
% ThetaHatDot3 = kTheta*Gamma3*(GStack(7:10,6*N+1:end)*...
%     (reshape(PStack(7:9,:),3*N,1)-GStack(7:10,6*N+1:end)'*ThetaHat3));
GammaDot = beta1*Gamma - kTheta*Gamma*...
    (GStack*GStack')/(1+alpha*norm((GStack*GStack')))*Gamma;
% GammaDot1 = beta1*Gamma1 - kTheta*Gamma1*...
%     (GStack(1:3,1:3*N)*GStack(1:3,1:3*N)')*Gamma1;
% GammaDot2 = beta1*Gamma2 - kTheta*Gamma2*...
%     (GStack(4:6,3*N+1:6*N)*GStack(4:6,3*N+1:6*N)')*Gamma2;
% GammaDot3 = beta1*Gamma3 - kTheta*Gamma3*...
%     (GStack(7:10,6*N+1:end)*GStack(7:10,6*N+1:end)')*Gamma3;
% ThetaHatDot = [ThetaHatDot1;ThetaHatDot2;ThetaHatDot3];
% GammaDot = [GammaDot1,zeros(3,7);
%          zeros(3,3),GammaDot2,zeros(3,4);
%          zeros(4,6),GammaDot3];
% GammaDot = beta1*Gamma - kTheta*(1/(1 + alpha*norm(GStack,2)))*Gamma*...
%     (GStack*GStack')*Gamma;

%Err = (reshape(CaligraphicFStack,n*N,1)-CaligraphicGStack'*ThetaStar);
ThetaTilde=ThetaStar(1:3,1)-ThetaHat;
%ThetaTilde=(reshape(CaligraphicFStack,n*N,1)-CaligraphicGStack'*ThetaStar);

% ThetaHatDot = persistThetaHatDot;

== matlab function Force_Att_Controller_Separated/Theta Update2 ==
  data: Gamma input; GammaDot output; ThetaHat input; GStack input; PStack input; N parameter; n parameter; m parameter; ThetaHatDot output; kTheta parameter; beta1 parameter; ThetaStar parameter; ThetaTilde output
function [GammaDot,ThetaHatDot,ThetaTilde]  = fcn(Gamma,ThetaHat,...
    GStack,PStack,N,n,m,kTheta, beta1, ThetaStar)
%#codegen
% persistent persistThetaHatDot
% if isempty(persistThetaHatDot)
%     persistThetaHatDot = zeros(10,1);
% end
%CaligraphicGStack is [CaligraphicG1' CaligraphicG2' ... CaligraphicGN']
%CaligraphicFStack is [CaligraphicF1 CaligraphicF2 ... CaligraphicFN]
alpha = 0.01;
% Gamma1 = Gamma(1:3,1:3);
% Gamma2 = Gamma(4:6,4:6);
% Gamma3 = Gamma(7:10,7:10);
% ThetaHat1 = ThetaHat(1:3,1);
% ThetaHat2 = ThetaHat(4:6,1);
% ThetaHat3 = ThetaHat(7:10,1);
ThetaHatDot = kTheta*Gamma*(GStack*...
    (reshape(PStack,n/3*N,1)-GStack'*ThetaHat));
% ThetaHatDot2 = kTheta*Gamma2*(GStack(4:6,3*N+1:6*N)*...
%     (reshape(PStack(4:6,:),3*N,1)-GStack(4:6,3*N+1:6*N)'*ThetaHat2));
% ThetaHatDot3 = kTheta*Gamma3*(GStack(7:10,6*N+1:end)*...
%     (reshape(PStack(7:9,:),3*N,1)-GStack(7:10,6*N+1:end)'*ThetaHat3));
GammaDot = beta1*Gamma - kTheta*Gamma*...
    (GStack*GStack')/(1+alpha*norm((GStack*GStack')))*Gamma;
% GammaDot1 = beta1*Gamma1 - kTheta*Gamma1*...
%     (GStack(1:3,1:3*N)*GStack(1:3,1:3*N)')*Gamma1;
% GammaDot2 = beta1*Gamma2 - kTheta*Gamma2*...
%     (GStack(4:6,3*N+1:6*N)*GStack(4:6,3*N+1:6*N)')*Gamma2;
% GammaDot3 = beta1*Gamma3 - kTheta*Gamma3*...
%     (GStack(7:10,6*N+1:end)*GStack(7:10,6*N+1:end)')*Gamma3;
% ThetaHatDot = [ThetaHatDot1;ThetaHatDot2;ThetaHatDot3];
% GammaDot = [GammaDot1,zeros(3,7);
%          zeros(3,3),GammaDot2,zeros(3,4);
%          zeros(4,6),GammaDot3];
% GammaDot = beta1*Gamma - kTheta*(1/(1 + alpha*norm(GStack,2)))*Gamma*...
%     (GStack*GStack')*Gamma;

%Err = (reshape(CaligraphicFStack,n*N,1)-CaligraphicGStack'*ThetaStar);
ThetaTilde=ThetaStar(4:6,1)-ThetaHat;
%ThetaTilde=(reshape(CaligraphicFStack,n*N,1)-CaligraphicGStack'*ThetaStar);

% ThetaHatDot = persistThetaHatDot;

== matlab function Force_Att_Controller_Separated/Generate Buffer3 ==
  settings: updateMethod=DISCRETE  sampleTime=Ts
  data: pbuff output; p input; u input; q input; qDot input; t input; T1 parameter; T2 parameter; Ts parameter; n parameter; L parameter; vecYTbuff output; P parameter
function [pbuff,vecYTbuff] = fcn(p,u,q,qDot,t,T1,T2,Ts,n,L,P)
%#codegen
persistent PTemp sigTemp;
if isempty(PTemp)
    PTemp = 0*ones(n/3,round((T1)/Ts)+1); % initalize the persistent variable
end

if isempty(sigTemp)
    sigTemp = zeros(n/3*(L+1),round((T1)/Ts)+1);
end
% Known part of the system dynamics
qDotbuff = zeros(9,1);
x1 = p(1:3,1);
x2 = p(4:6,1);
xc = p(7:9,1);
x1Dot = q(1:3,1);
x2Dot = q(4:6,1);
xcDot = q(7:9,1);
m1 = P.m;
m2 = m1;
Mc = P.Mc;
g = P.g;
k = P.k;

e3 = [0 0 1]';

R_theta = eye(3,3);     

r1 = [0 -0.15 0]';
r2 = [0 0.15 0]';

a1 = xc + R_theta*r1; 

a2 = xc + R_theta*r2;

z1 = x1 - a1;

z2 = x2 - a2;

f1 = k*z1;  % linear model 

f2 = k*z2;   % linear model 


fo = [(f1 + f2)];

Y_N = diag([1/m1*norm(x1Dot)*x1Dot;
             1/m2*norm(x2Dot)*x2Dot]);
Y_c = [eye(3),qDot(7:9,1) + g*e3];


Y = [Y_c];
 
qDotbuff(1:6,1) = qDot(1:6,1);
qDotbuff(7:9,1) = zeros(3,1);

sig = reshape(Y.',n/3*(L+1),1);

PPP=PTemp(:,2:end);
SSS=sigTemp(:,2:end);
PTemp=[PPP fo];
sigTemp=[SSS sig];
pbuff=PTemp;
vecYTbuff=sigTemp;

== matlab function Force_Att_Controller_Separated/Generate Affine System3 ==
  data: P output; pbuff input; vecYTbuff input; t input; Ts parameter; T2 parameter; T1 parameter; vecTGHat output
function [P,vecTGHat]  = fcn(pbuff,vecYTbuff,t ,Ts, T2, T1)
%#codegen
T1Round=round(T1/Ts);

P1=pbuff(:,end-T1Round:end);
G1=vecYTbuff(:,end-T1Round:end);

P = (t>T1)*Ts*trapz(P1,2);
vecTGHat = (t>T1)*Ts*trapz(G1,2);

== matlab function Force_Att_Controller_Separated/History Stack3 ==
  settings: updateMethod=DISCRETE  sampleTime=Ts
  data: P input; GTStack output; vecTG input; N parameter; n parameter; L parameter; PStack output; nPoint output; CurrentSVD output
function [GTStack,PStack,nPoint,CurrentSVD] =...
    fcn(P,vecTG, N, n, L )
%#codegen,FStackStored, GStackStored, PStackStored
persistent GStackHPersist PStackHPersist nPoints eta;
% if isempty(FStackHPersist)
% %    FStackHPersist = FStackStored; % initalize the persistent variable
%      FStackHPersist = zeros(n,N);
% end
if isempty(GStackHPersist)
 %   GStackHPersist = GStackStored;
    GStackHPersist = zeros(L+1,n/3*N);
end
if isempty(PStackHPersist)
%    PStackHPersist = PStackStored;
     PStackHPersist = zeros(n/3,N);
end
if isempty(nPoints)
    nPoints = 0;
end
if isempty(eta)
    eta = 0;
end
%GHatTStack is [intY1' intY2' ... intYN']
%FHatStack is [FHat1 FHat2 ... FHatN]
%and so is PStack
G = (reshape(vecTG,L+1,n/3)).';

%Operations 
CurrentScriptH = GStackHPersist*GStackHPersist';
CurrentSingularValue = min(svd(CurrentScriptH));
SingularValueList = zeros(N,1);
for i=1:N
    ithGTranspose = GStackHPersist(:,(i-1)*n/3+1:i*n/3);
    NewScriptH = CurrentScriptH + G'*G...
        -ithGTranspose*ithGTranspose';
    SingularValueList(i,1)=min(svd(NewScriptH));
end

[NewSingularValue,ind]=max(SingularValueList);
%Update persistent variables
if NewSingularValue>CurrentSingularValue + 0*CurrentSingularValue
    GStackHPersist(:,(ind-1)*n/3+1:ind*n/3) = G';
    %FStackHPersist(:,ind) = FHat;
    PStackHPersist(:,ind) = P;
    nPoints = nPoints+1;
end
if NewSingularValue>eta
    eta=NewSingularValue;
end
%Output
CurrentSVD = min(svd(GStackHPersist*GStackHPersist'));
%FStack=FStackHPersist;
GTStack=GStackHPersist;
PStack=PStackHPersist;
nPoint = nPoints;



% 

% 
% 
% persistent FStackHPersist GStackHPersist PStackHPersist FStackGPersist GStackGPersist PStackGPersist nPoints nPurges eta;
% if isempty(FStackHPersist)
%     FStackHPersist = zeros(n,N); % initalize the persistent variable
% end
% if isempty(GStackHPersist)
%     GStackHPersist = zeros(L,n*N);
% end
% if isempty(PStackHPersist)
%     PStackHPersist = zeros(n,N);
% end
% if isempty(FStackGPersist)
%     FStackGPersist = zeros(n,N); % initalize the persistent variable
% end
% if isempty(GStackGPersist)
%     GStackGPersist = zeros(L,n*N);
% end
% if isempty(PStackGPersist)
%     PStackGPersist = zeros(n,N);
% end
% if isempty(nPoints)
%     nPoints = 0;
% end
% if isempty(nPurges)
%     nPurges = 0;
% end
% if isempty(eta)
%     eta = 0;
% end
% %GHatTStack is [intY1' intY2' ... intYN']
% %FHatStack is [FHat1 FHat2 ... FHatN]
% %and so is PStack
% GHat = (reshape(vecTG,L,n)).';
% 
% %Operations 
% CurrentScriptG = GStackGPersist*GStackGPersist';
% CurrentSingularValue = min(svd(CurrentScriptG));
% SingularValueList = zeros(N,1);
% for i=1:N
%     ithGTranspose = GStackGPersist(:,(i-1)*n+1:i*n);
%     NewScriptG = CurrentScriptG + GHat'*GHat...
%         -ithGTranspose*ithGTranspose';
%     SingularValueList(i,1)=min(svd(NewScriptG));
% end
% [NewSingularValue,ind]=max(SingularValueList);
% %Update persistent variables
% if NewSingularValue>CurrentSingularValue + 0*CurrentSingularValue
%     GStackGPersist(:,(ind-1)*n+1:ind*n) = GHat';
%     FStackGPersist(:,ind) = FHat;
%     PStackGPersist(:,ind) = P;
%     nPoints = nPoints+1;
% end
% if nPurges==0
%     FStackHPersist=FStackGPersist;
% end
% if nPoints >= N && NewSingularValue>0.95*eta
%     nPoints = 0;
%     FStackHPersist = FStackGPersist;
%     FStackGPersist = zeros(n,N);
%     GStackHPersist = GStackGPersist;
%     GStackGPersist = zeros(L,n*N);
%     PStackHPersist = PStackGPersist;
%     PStackGPersist = zeros(n,N);
%     nPurges = nPurges+1;
% end
% if NewSingularValue>eta
%     eta=NewSingularValue;
% end
% %Output
% CurrentSVD = min(svd(GStackHPersist*GStackHPersist'));
% FStack=FStackHPersist;
% GTStack=GStackHPersist;
% PStack=PStackHPersist;
% nPoint = nPoints;
% nPurge = nPurges;

== matlab function Force_Att_Controller_Separated/Theta Update3 ==
  data: Gamma input; GammaDot output; ThetaHat input; GStack input; PStack input; N parameter; n parameter; m parameter; ThetaHatDot output; kTheta parameter; beta1 parameter; ThetaStar parameter; ThetaTilde output
function [GammaDot,ThetaHatDot,ThetaTilde]  = fcn(Gamma,ThetaHat,...
    GStack,PStack,N,n,m,kTheta, beta1, ThetaStar)
%#codegen
% persistent persistThetaHatDot
% if isempty(persistThetaHatDot)
%     persistThetaHatDot = zeros(10,1);
% end
%CaligraphicGStack is [CaligraphicG1' CaligraphicG2' ... CaligraphicGN']
%CaligraphicFStack is [CaligraphicF1 CaligraphicF2 ... CaligraphicFN]
alpha = 0.01;
% Gamma1 = Gamma(1:3,1:3);
% Gamma2 = Gamma(4:6,4:6);
% Gamma3 = Gamma(7:10,7:10);
% ThetaHat1 = ThetaHat(1:3,1);
% ThetaHat2 = ThetaHat(4:6,1);
% ThetaHat3 = ThetaHat(7:10,1);
ThetaHatDot = kTheta*Gamma*(GStack*...
    (reshape(PStack,n/3*N,1)-GStack'*ThetaHat));
% ThetaHatDot2 = kTheta*Gamma2*(GStack(4:6,3*N+1:6*N)*...
%     (reshape(PStack(4:6,:),3*N,1)-GStack(4:6,3*N+1:6*N)'*ThetaHat2));
% ThetaHatDot3 = kTheta*Gamma3*(GStack(7:10,6*N+1:end)*...
%     (reshape(PStack(7:9,:),3*N,1)-GStack(7:10,6*N+1:end)'*ThetaHat3));
GammaDot = beta1*Gamma - kTheta*Gamma*...
    (GStack*GStack')/(1+alpha*norm((GStack*GStack')))*Gamma;
% GammaDot1 = beta1*Gamma1 - kTheta*Gamma1*...
%     (GStack(1:3,1:3*N)*GStack(1:3,1:3*N)')*Gamma1;
% GammaDot2 = beta1*Gamma2 - kTheta*Gamma2*...
%     (GStack(4:6,3*N+1:6*N)*GStack(4:6,3*N+1:6*N)')*Gamma2;
% GammaDot3 = beta1*Gamma3 - kTheta*Gamma3*...
%     (GStack(7:10,6*N+1:end)*GStack(7:10,6*N+1:end)')*Gamma3;
% ThetaHatDot = [ThetaHatDot1;ThetaHatDot2;ThetaHatDot3];
% GammaDot = [GammaDot1,zeros(3,7);
%          zeros(3,3),GammaDot2,zeros(3,4);
%          zeros(4,6),GammaDot3];
% GammaDot = beta1*Gamma - kTheta*(1/(1 + alpha*norm(GStack,2)))*Gamma*...
%     (GStack*GStack')*Gamma;

%Err = (reshape(CaligraphicFStack,n*N,1)-CaligraphicGStack'*ThetaStar);
ThetaTilde=ThetaStar(7:10,1)-ThetaHat;
%ThetaTilde=(reshape(CaligraphicFStack,n*N,1)-CaligraphicGStack'*ThetaStar);

% ThetaHatDot = persistThetaHatDot;

== matlab function Force_Att_Controller_Separated/Theta Update4 ==
  data: ThetaHat output; Gamma1 input; Gamma output; ThetaHat1 input; Gamma2 input; ThetaHat2 input; Gamma3 input; ThetaHat3 input
function [ThetaHat,Gamma]  = fcn(Gamma1,ThetaHat1,Gamma2,ThetaHat2,Gamma3,ThetaHat3)
%#codegen
% persistent persistThetaHatDot
% if isempty(persistThetaHatDot)
%     persistThetaHatDot = zeros(10,1);
% end
%CaligraphicGStack is [CaligraphicG1' CaligraphicG2' ... CaligraphicGN']
%CaligraphicFStack is [CaligraphicF1 CaligraphicF2 ... CaligraphicFN]
% alpha = 0;
% Gamma1 = Gamma(1:3,1:3);
% Gamma2 = Gamma(4:6,4:6);
% Gamma3 = Gamma(7:10,7:10);
% ThetaHat1 = ThetaHat(1:3,1);
% ThetaHat2 = ThetaHat(4:6,1);
% ThetaHat3 = ThetaHat(7:10,1);
% ThetaHatDot = kTheta*Gamma*(GStack*...
%     (reshape(PStack,n/3*N,1)-GStack'*ThetaHat));
% ThetaHatDot2 = kTheta*Gamma2*(GStack(4:6,3*N+1:6*N)*...
%     (reshape(PStack(4:6,:),3*N,1)-GStack(4:6,3*N+1:6*N)'*ThetaHat2));
% ThetaHatDot3 = kTheta*Gamma3*(GStack(7:10,6*N+1:end)*...
%     (reshape(PStack(7:9,:),3*N,1)-GStack(7:10,6*N+1:end)'*ThetaHat3));
% GammaDot = beta1*Gamma - kTheta*Gamma*...
%     (GStack*GStack')/(1+alpha*norm((GStack*GStack')))*Gamma;
% GammaDot1 = beta1*Gamma1 - kTheta*Gamma1*...
%     (GStack(1:3,1:3*N)*GStack(1:3,1:3*N)')*Gamma1;
% GammaDot2 = beta1*Gamma2 - kTheta*Gamma2*...
%     (GStack(4:6,3*N+1:6*N)*GStack(4:6,3*N+1:6*N)')*Gamma2;
% GammaDot3 = beta1*Gamma3 - kTheta*Gamma3*...
%     (GStack(7:10,6*N+1:end)*GStack(7:10,6*N+1:end)')*Gamma3;
ThetaHat = [ThetaHat1;ThetaHat2;ThetaHat3];
Gamma = [Gamma1,zeros(3,7);
         zeros(3,3),Gamma2,zeros(3,4);
         zeros(4,6),Gamma3];
% GammaDot = beta1*Gamma - kTheta*(1/(1 + alpha*norm(GStack,2)))*Gamma*...
%     (GStack*GStack')*Gamma;

%Err = (reshape(CaligraphicFStack,n*N,1)-CaligraphicGStack'*ThetaStar);
% ThetaTilde=ThetaStar(4:6,1)-ThetaHat;
%ThetaTilde=(reshape(CaligraphicFStack,n*N,1)-CaligraphicGStack'*ThetaStar);

% ThetaHatDot = persistThetaHatDot;

== matlab function Force_Att_Controller_Separated/Subsystem/Quadrotor1/Att Controller ==
  data: x input; u output; desired input; prev_x input; P parameter
function u = fcn(x, desired, prev_x, P)
%#codegen
% Reference: A Simple Attitude Control of Quadrotor Helicopter Based on
%Ziegler-Nichols Rules for Tuning PD Parameters

%ZeFang He and Long Zhao

u = zeros(4,1);
%timestep size
Ts = P.Ts;

L = P.L;  Ix = P.Ix;  Iy = P.Iy;  Iz = P.Iz; m = P.m; g = P.g;
b1 = 1/Ix;
b2 = 1/Iy;
b3 = 1/Iz;

a1 = (Iy-Iz)/Ix;
a3 = (Iz-Ix)/Iy;
a5 = (Ix-Iy)/Iz;

K2 = P.K2;
K3 = P.K3;
K4 = P.K4;

Kp2 = P.Kp2;
Kp3 = P.Kp3;
Kp4 = P.Kp4;

Kd2 = P.Kd2;
Kd3 = P.Kd3;
Kd4 = P.Kd4;


err2 = (desired(1) - x(1));
err3 = (desired(2) - x(2));
err4 = (desired(3) - x(3));
prev_err2 = (desired(1) - prev_x(1));
prev_err3 = (desired(2) - prev_x(2));
prev_err4 = (desired(3) - prev_x(3));


u(1) = 10;
u(2) = 1/b1*(K2*x(4)-a1*x(5)*x(6)) + Kp2*err2 + Kd2*(err2-prev_err2)/Ts;
u(3) = 1/b2*(K3*x(5)-a3*x(4)*x(6)) + Kp3*err3 + Kd3*(err3-prev_err3)/Ts;
u(4) = 1/b3*(K4*x(6)-a5*x(4)*x(5)) + Kp4*err4 + Kd4*(err4-prev_err4)/Ts;

== matlab function Force_Att_Controller_Separated/Subsystem/Quadrotor2/Att Controller ==
  data: x input; u output; desired input; prev_x input; P parameter
function u = fcn(x, desired, prev_x, P)
%#codegen
% Reference: A Simple Attitude Control of Quadrotor Helicopter Based on
%Ziegler-Nichols Rules for Tuning PD Parameters

%ZeFang He and Long Zhao

u = zeros(4,1);
%timestep size
Ts = P.Ts;

L = P.L;  Ix = P.Ix;  Iy = P.Iy;  Iz = P.Iz; m = P.m; g = P.g;
b1 = 1/Ix;
b2 = 1/Iy;
b3 = 1/Iz;

a1 = (Iy-Iz)/Ix;
a3 = (Iz-Ix)/Iy;
a5 = (Ix-Iy)/Iz;

K2 = P.K2;
K3 = P.K3;
K4 = P.K4;

Kp2 = P.Kp2;
Kp3 = P.Kp3;
Kp4 = P.Kp4;

Kd2 = P.Kd2;
Kd3 = P.Kd3;
Kd4 = P.Kd4;


err2 = (desired(1) - x(1));
err3 = (desired(2) - x(2));
err4 = (desired(3) - x(3));
prev_err2 = (desired(1) - prev_x(1));
prev_err3 = (desired(2) - prev_x(2));
prev_err4 = (desired(3) - prev_x(3));


u(1) = 10;
u(2) = 1/b1*(K2*x(4)-a1*x(5)*x(6)) + Kp2*err2 + Kd2*(err2-prev_err2)/Ts;
u(3) = 1/b2*(K3*x(5)-a3*x(4)*x(6)) + Kp3*err3 + Kd3*(err3-prev_err3)/Ts;
u(4) = 1/b3*(K4*x(6)-a5*x(4)*x(5)) + Kp4*err4 + Kd4*(err4-prev_err4)/Ts;
